simulink model "igct_diode"  (R2023b)
settings: Solver=VariableStepAuto  StartTime=0.0  StopTime=10.0  RelTol=1e-3
values from neighbouring files (symbols this model uses):
  temp_init = 40    [power_sysinit.m]
  Ts1 = 1e-6    (= 1e-06)    [power_sysinit.m]
  Ts2 = 500E-6    (= 0.0005)    [power_sysinit.m]
  Udc = 2500    [power_sysinit.m]
undefined symbols (not defined in the file or in its folder): DIODE_204520, DIODE_344520, DIODE_364520, DIODE_364521, DIODE_D1031SH, DIODE_D1331SH, IGCT_364520_36, IGCT_364521_36, IGCT_654522_6, magnitude, Rch_DIODE, Rch_tau_DIODE, Rjc1_DIODE, Rjc1_tau_DIODE, Rjc2_DIODE, Rjc2_tau_DIODE, Rjc3_DIODE, Rjc3_tau_DIODE, Rth_h, Rth_h_tau
libraries: spsMeanLib x304, simulink x52, spsRMSLib x52
(part 7 of 11)

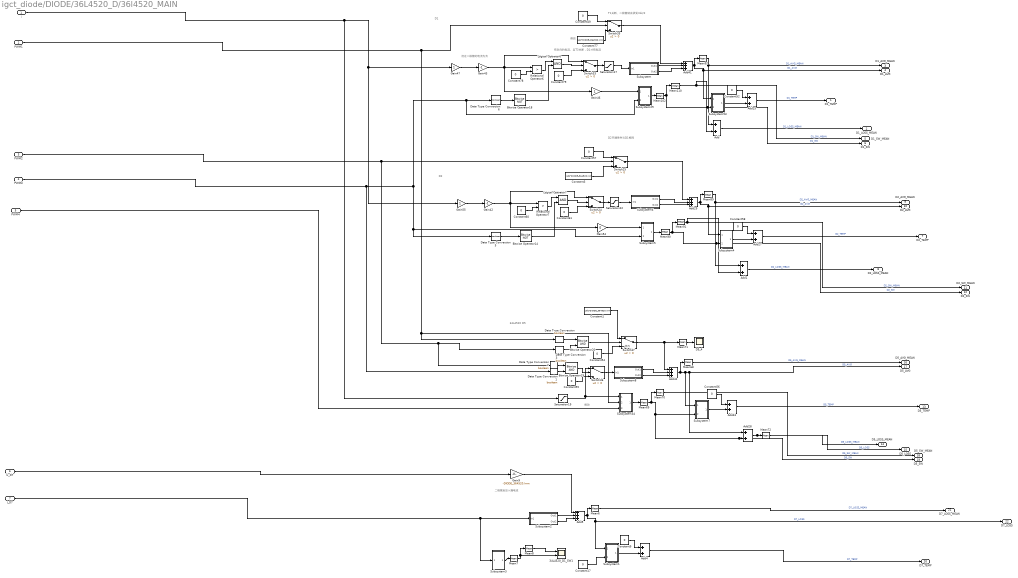
== system igct_diode/DIODE/36L4520_D/36l4520_MAIN ==
  note: 修改
  note: 34L4520 D5
  note: 修改
  note: 二极管反压×漏电流
  note: D2
  note: 有负向的电流、且T3关断，D1才有电流
  note: 修改
  note: 流过二极管的电流为负
  note: D2开通条件与D1相同
  note: T1关断、二极管就会承受Vdc/2
  note: D1
  i : Inport
  PWM1 : Inport  Port=2
  PWM2 : Inport  Port=3
  PWM3 : Inport  Port=4
  PWM4 : Inport  Port=5
  U_D7 : Inport  Port=6
  I_D7 : Inport  Port=7
  34L4520_D1_SW1 : Scope  NumInputPorts=2
  Add{,1,4,25,27..28,43} (7 alike) : Sum
  Add{5,29,41..42} (4 alike) : Sum  Inputs=+++
  Bitwise Operator14 : simulink/Logic and Bit Operations/Bitwise Operator  logicop=NOT  UseBitMask=off  BitMask=bin2dec('11011001')  BitMaskRealWorld=Stored Integer
  Bitwise Operator18 : simulink/Logic and Bit Operations/Bitwise Operator  logicop=NOT  UseBitMask=off  BitMask=bin2dec('11011001')  BitMaskRealWorld=Stored Integer
  Bitwise Operator19 : simulink/Logic and Bit Operations/Bitwise Operator  logicop=AND  UseBitMask=off  NumInputPorts=2  BitMask=bin2dec('11011001')  BitMaskRealWorld=Stored Integer
  Bitwise Operator20 : simulink/Logic and Bit Operations/Bitwise Operator  logicop=AND  UseBitMask=off  NumInputPorts=2  BitMask=bin2dec('11011001')  BitMaskRealWorld=Stored Integer
  Constant1 : Constant  Value=Udc*DIODE_364520.Irrm
  Constant{9,17,49,52,54..58,60..61,78..79} (13 alike) : Constant  Value=0
  Constant3 : Constant  Value=Udc*DIODE_364520.Irrm
  Constant77 : Constant  Value=Udc*DIODE_364520.Irrm
  D5_4 : Scope
  Data Type Conversion{,1..3,5..6} (6 alike) : DataTypeConversion  OutDataTypeStr=boolean  SaturateOnIntegerOverflow=off  RndMeth=Floor
  Gain42 : Gain  Gain=-1
  Gain43 : Gain  Gain=-1
  Gain46 : Gain
  Gain47 : Gain
  Gain54 : Gain  Gain=0
  Gain55 : Gain
  Gain9 : Gain  Gain=-DIODE_364520.Irrm
  Logical Operator6 : Logic  AllPortsSameDT=off  OutDataTypeStr=boolean
  Logical Operator7 : Logic  AllPortsSameDT=off  OutDataTypeStr=boolean
  Mean{7,69,90,102} (4 alike) : spsMeanLib/Mean  Freq=2000  Vinit=0  Ts=Ts1
  Mean{6,8,68,70,72,91..92,110} (8 alike) : spsMeanLib/Mean  Freq=f  Vinit=0  Ts=Ts1
  Mean71 : spsMeanLib/Mean  Freq=1  Vinit=0  Ts=Ts1
  Mean89 : spsMeanLib/Mean  Freq=f  Vinit=0  Ts=1e-6
  Relational Operator6 : RelationalOperator  Operator=>  OutDataTypeStr=boolean  RndMeth=Simplest  InputSameDT=off
  Relational Operator7 : RelationalOperator  Operator=>  OutDataTypeStr=boolean  RndMeth=Simplest  InputSameDT=off
  Saturation17 : Saturate  UpperLimit=5500  LowerLimit=0
  Saturation19 : Saturate  UpperLimit=5000  LowerLimit=0
  Saturation22 : Saturate  UpperLimit=5500  LowerLimit=0
  Subsystem : Subsystem
  Subsystem1 : Subsystem
  Subsystem2 : Subsystem
  Subsystem29 : Subsystem
  Subsystem3 : Subsystem
  Subsystem34 : Subsystem
  Subsystem4 : Subsystem
  Subsystem5 : Subsystem
  Subsystem53 : Subsystem
  Subsystem6 : Subsystem
  Subsystem7 : Subsystem
  Subsystem8 : Subsystem
  Switch{24..25,33,35..37} (6 alike) : Switch  Criteria=u2 > Threshold  SaturateOnIntegerOverflow=off  InputSameDT=off
  D1_TEMP : Outport
  D1_LOSS_MEAN : Outport  Port=2
  D1_AVG_MEAN : Outport  Port=3
  D1_AVG : Outport  Port=4
  D1_SW_MEAN : Outport  Port=5
  D1_SW : Outport  Port=6
  D2_TEMP : Outport  Port=7
  D2_LOSS_MEAN : Outport  Port=8
  D2_AVG_MEAN : Outport  Port=9
  D2_AVG : Outport  Port=10
  D2_SW_MEAN : Outport  Port=11
  D2_SW : Outport  Port=12
  D5_TEMP : Outport  Port=13
  D5_LOSS_MEAN : Outport  Port=14
  D5_LOSS : Outport  Port=15
  D5_AVG_MEAN : Outport  Port=16
  D5_AVG : Outport  Port=17
  D5_SW_MEAN : Outport  Port=18
  D5_SW : Outport  Port=19
  D7_TEMP : Outport  Port=20
  D7_LOSS_MEAN : Outport  Port=21
  D7_LOSS : Outport  Port=22
  wires:
  Add1/1 -> D2_LOSS_MEAN/1  "D2_LOSS_MEAN"
  Add/1 -> D1_LOSS_MEAN/1  "D1_LOSS_MEAN"
  Add27/1 -> D2_TEMP/1  "D2_TEMP"
  Add4/1 -> D7_TEMP/1  "D7_TEMP"
  U_D7/1 -> Gain9/1
  Mean70/1 -> D5_SW_MEAN/1  "D5_SW_MEAN"
  Subsystem/2(Out2) -> Add41/3
  Saturation17/1 -> Subsystem/1(In1)
  Constant60/1 -> Relational Operator7/2
  Gain47/1 -> Gain43/1
  Data Type Conversion6/1 -> Bitwise Operator18/1
  Constant78/1 -> Relational Operator6/2
  Data Type Conversion5/1 -> Bitwise Operator14/1
  Constant57/1 -> Switch25/1
  Bitwise Operator18/1 -> Logical Operator6/2
  Constant77/1 -> Switch35/3
  Mean89/1 -> Add1/1, D2_AVG_MEAN/1  "D2_AVG_MEAN"
  Subsystem53/1(Out1) -> Add25/2
  Constant52/1 -> Add25/1
  Add43/1 -> D5_TEMP/1  "D5_TEMP"
  Logical Operator6/1 -> Switch33/2
  Constant49/1 -> Switch35/1
  Gain46/1 -> Subsystem29/1(In1)
  Gain42/1 -> Switch24/1, Gain54/1, Relational Operator7/1
  Switch24/1 -> Saturation22/1
  Constant79/1 -> Switch33/3
  Mean92/1 -> Add/1, D1_AVG_MEAN/1  "D1_AVG_MEAN"
  Switch35/1 -> Add41/1
  Switch25/1 -> Add29/1
  Mean6/1 -> D7_LOSS_MEAN/1  "D7_LOSS_MEAN"
  Gain43/1 -> Relational Operator6/1, Gain46/1, Switch33/1
  Add41/1 -> Mean92/1, Subsystem53/1(In1), D1_AVG/1  "D1_AVG"
  Subsystem4/1(Out1) -> Add27/2
  Data Type Conversion2/1 -> Bitwise Operator19/1
  Constant55/1 -> Switch36/3
  Subsystem3/1(Out1) -> Mean7/1
  Subsystem6/2(Out2) -> Add29/3
  Switch37/1 -> Add42/1, Mean71/1
  Constant54/1 -> Switch37/3
  Subsystem7/1(Out1) -> Add43/2
  Subsystem/1(Out1) -> Add41/2
  Gain9/1 -> Add5/1
  Constant58/1 -> Add27/1
  Subsystem8/1(Out1) -> Add42/2
  Mean8/1 -> 34L4520_D1_SW1/1
  Gain54/1 -> Subsystem5/1(In1)
  Mean102/1 -> Subsystem53/2(In2), D1_SW/1, Mean110/1  "D1_SW"
  Subsystem1/1(Out1) -> Add4/2
  Subsystem5/1(Out1) -> Mean90/1
  I_D7/1 -> Subsystem2/1(In1), Subsystem3/1(In1)
  Logical Operator7/1 -> Switch24/2
  Add5/1 -> Subsystem1/1(In1), D7_LOSS/1, Mean6/1  "D7_LOSS"
  Data Type Conversion3/1 -> Bitwise Operator20/2
  Mean7/1 -> Mean8/1, 34L4520_D1_SW1/2
  Relational Operator7/1 -> Logical Operator7/1
  Constant17/1 -> Subsystem1/2(In2)
  Subsystem2/2(Out2) -> Add5/3
  Add25/1 -> D1_TEMP/1  "D1_TEMP"
  Mean69/1 -> Mean70/1, Subsystem7/2(In2), Add28/2, D5_SW/1  "D5_SW"
  Bitwise Operator20/1 -> Switch37/2
  PWM4/1 -> Subsystem34/3(In3)
  Bitwise Operator19/1 -> Switch36/2
  Mean91/1 -> Add1/2, D2_SW_MEAN/1  "D2_SW_MEAN"
  PWM2/1 -> Switch25/2, Data Type Conversion3/1, Data Type Conversion2/1
  Switch33/1 -> Saturation17/1
  Mean110/1 -> Add/2, D1_SW_MEAN/1  "D1_SW_MEAN"
  Mean71/1 -> D5_4/1
  PWM3/1 -> Subsystem5/2(In2), Data Type Conversion5/1, Subsystem29/2(In2), Data Type Conversion6/1, Data Type Conversion1/1
  i/1 -> Gain47/1, Gain55/1, Saturation19/1
  Subsystem6/1(Out1) -> Add29/2
  Data Type Conversion1/1 -> Bitwise Operator19/2
  Constant61/1 -> Switch24/3
  Mean72/1 -> D5_LOSS_MEAN/1  "D5_LOSS_MEAN"
  Mean90/1 -> Mean91/1, D2_SW/1, Subsystem4/2(In2)  "D2_SW"
  PWM1/1 -> Switch35/2, Data Type Conversion/1, Subsystem34/2(In2)
  Relational Operator6/1 -> Logical Operator6/1
  Mean68/1 -> D5_AVG_MEAN/1  "D5_AVG_MEAN"
  Saturation19/1 -> Subsystem34/1(In1), Switch36/1
  Switch36/1 -> Subsystem8/1(In1)
  Subsystem8/2(Out2) -> Add42/3
  Gain55/1 -> Gain42/1
  Constant3/1 -> Switch25/3
  Constant9/1 -> Add4/1
  Subsystem34/1(Out1) -> Mean69/1
  Add42/1 -> Mean68/1, Subsystem7/1(In1), Add28/1, D5_AVG/1  "D5_AVG"
  Data Type Conversion/1 -> Bitwise Operator20/1
  Bitwise Operator14/1 -> Logical Operator7/2
  Saturation22/1 -> Subsystem6/1(In1)
  Add29/1 -> Subsystem4/1(In1), D2_AVG/1, Mean89/1  "D2_AVG"
  Constant1/1 -> Switch37/1
  Constant56/1 -> Add43/1
  Subsystem2/1(Out1) -> Add5/2
  Subsystem29/1(Out1) -> Mean102/1
  Add28/1 -> Mean72/1, D5_LOSS/1  "D5_LOSS"

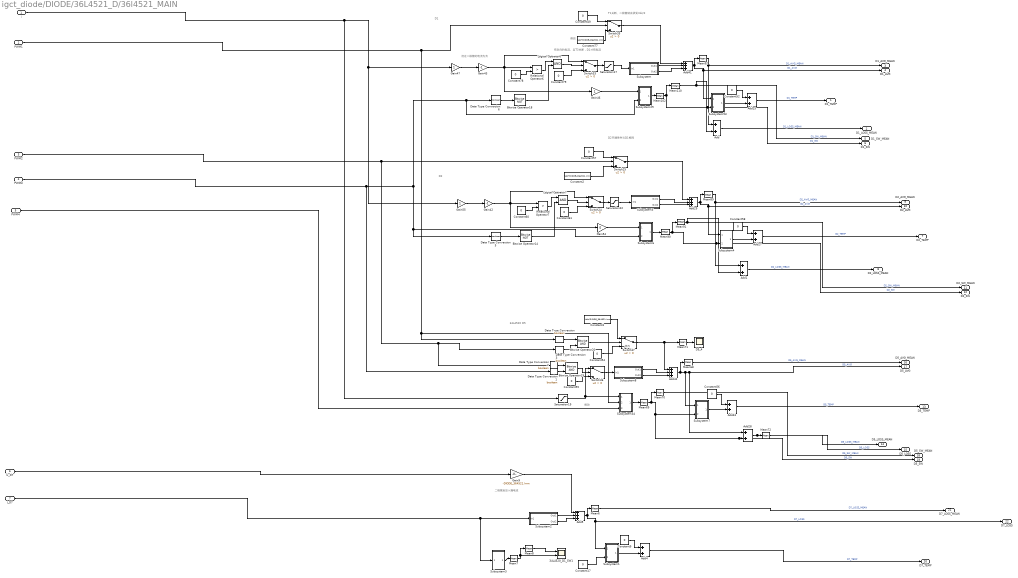
== system igct_diode/DIODE/36L4521_D/36l4521_MAIN ==
  note: D1
  note: T1关断、二极管就会承受Vdc/2
  note: D2开通条件与D1相同
  note: 流过二极管的电流为负
  note: 修改
  note: 有负向的电流、且T3关断，D1才有电流
  note: D2
  note: 二极管反压×漏电流
  note: 修改
  note: 34L4520 D5
  note: 修改
  i : Inport
  PWM1 : Inport  Port=2
  PWM2 : Inport  Port=3
  PWM3 : Inport  Port=4
  PWM4 : Inport  Port=5
  U_D7 : Inport  Port=6
  I_D7 : Inport  Port=7
  34L4520_D1_SW1 : Scope  NumInputPorts=2
  Add{,1,4,25,27..28,43} (7 alike) : Sum
  Add{5,29,41..42} (4 alike) : Sum  Inputs=+++
  Bitwise Operator14 : simulink/Logic and Bit Operations/Bitwise Operator  logicop=NOT  UseBitMask=off  BitMask=bin2dec('11011001')  BitMaskRealWorld=Stored Integer
  Bitwise Operator18 : simulink/Logic and Bit Operations/Bitwise Operator  logicop=NOT  UseBitMask=off  BitMask=bin2dec('11011001')  BitMaskRealWorld=Stored Integer
  Bitwise Operator19 : simulink/Logic and Bit Operations/Bitwise Operator  logicop=AND  UseBitMask=off  NumInputPorts=2  BitMask=bin2dec('11011001')  BitMaskRealWorld=Stored Integer
  Bitwise Operator20 : simulink/Logic and Bit Operations/Bitwise Operator  logicop=AND  UseBitMask=off  NumInputPorts=2  BitMask=bin2dec('11011001')  BitMaskRealWorld=Stored Integer
  Constant{9,17,49,52,54..58,60..61,78..79} (13 alike) : Constant  Value=0
  Constant2 : Constant  Value=Udc*DIODE_364521.Irrm
  Constant3 : Constant  Value=Udc*DIODE_364521.Irrm
  Constant77 : Constant  Value=Udc*DIODE_364521.Irrm
  D5_4 : Scope
  Data Type Conversion{,1..3,5..6} (6 alike) : DataTypeConversion  OutDataTypeStr=boolean  SaturateOnIntegerOverflow=off  RndMeth=Floor
  Gain42 : Gain  Gain=-1
  Gain43 : Gain  Gain=-1
  Gain46 : Gain
  Gain47 : Gain
  Gain54 : Gain  Gain=0
  Gain55 : Gain
  Gain9 : Gain  Gain=-DIODE_364521.Irrm
  Logical Operator6 : Logic  AllPortsSameDT=off  OutDataTypeStr=boolean
  Logical Operator7 : Logic  AllPortsSameDT=off  OutDataTypeStr=boolean
  Mean{7,69,90,102} (4 alike) : spsMeanLib/Mean  Freq=2000  Vinit=0  Ts=Ts1
  Mean{6,8,68,70,72,91..92,110} (8 alike) : spsMeanLib/Mean  Freq=f  Vinit=0  Ts=Ts1
  Mean71 : spsMeanLib/Mean  Freq=1  Vinit=0  Ts=Ts1
  Mean89 : spsMeanLib/Mean  Freq=f  Vinit=0  Ts=1e-6
  Relational Operator6 : RelationalOperator  Operator=>  OutDataTypeStr=boolean  RndMeth=Simplest  InputSameDT=off
  Relational Operator7 : RelationalOperator  Operator=>  OutDataTypeStr=boolean  RndMeth=Simplest  InputSameDT=off
  Saturation17 : Saturate  UpperLimit=5500  LowerLimit=0
  Saturation19 : Saturate  UpperLimit=5000  LowerLimit=0
  Saturation22 : Saturate  UpperLimit=5500  LowerLimit=0
  Subsystem : Subsystem
  Subsystem1 : Subsystem
  Subsystem2 : Subsystem
  Subsystem29 : Subsystem
  Subsystem3 : Subsystem
  Subsystem34 : Subsystem
  Subsystem4 : Subsystem
  Subsystem5 : Subsystem
  Subsystem53 : Subsystem
  Subsystem6 : Subsystem
  Subsystem7 : Subsystem
  Subsystem8 : Subsystem
  Switch{24..25,33,35..37} (6 alike) : Switch  Criteria=u2 > Threshold  SaturateOnIntegerOverflow=off  InputSameDT=off
  D1_TEMP : Outport
  D1_LOSS_MEAN : Outport  Port=2
  D1_AVG_MEAN : Outport  Port=3
  D1_AVG : Outport  Port=4
  D1_SW_MEAN : Outport  Port=5
  D1_SW : Outport  Port=6
  D2_TEMP : Outport  Port=7
  D2_LOSS_MEAN : Outport  Port=8
  D2_AVG_MEAN : Outport  Port=9
  D2_AVG : Outport  Port=10
  D2_SW_MEAN : Outport  Port=11
  D2_SW : Outport  Port=12
  D5_TEMP : Outport  Port=13
  D5_LOSS_MEAN : Outport  Port=14
  D5_LOSS : Outport  Port=15
  D5_AVG_MEAN : Outport  Port=16
  D5_AVG : Outport  Port=17
  D5_SW_MEAN : Outport  Port=18
  D5_SW : Outport  Port=19
  D7_TEMP : Outport  Port=20
  D7_LOSS_MEAN : Outport  Port=21
  D7_LOSS : Outport  Port=22
  wires:
  Add28/1 -> D5_LOSS/1, Mean72/1  "D5_LOSS"
  Subsystem29/1(Out1) -> Mean102/1
  Subsystem2/1(Out1) -> Add5/2
  Constant56/1 -> Add43/1
  Constant3/1 -> Switch37/1
  Add29/1 -> Mean89/1, Subsystem4/1(In1), D2_AVG/1  "D2_AVG"
  Saturation22/1 -> Subsystem5/1(In1)
  Bitwise Operator14/1 -> Logical Operator7/2
  Data Type Conversion/1 -> Bitwise Operator20/1
  Add42/1 -> Subsystem7/1(In1), D5_AVG/1, Add28/1, Mean68/1  "D5_AVG"
  Subsystem34/1(Out1) -> Mean69/1
  Constant9/1 -> Add4/1
  Constant2/1 -> Switch25/3
  Gain55/1 -> Gain42/1
  Subsystem8/2(Out2) -> Add42/3
  Switch36/1 -> Subsystem8/1(In1)
  Saturation19/1 -> Switch36/1, Subsystem34/1(In1)
  Mean68/1 -> D5_AVG_MEAN/1  "D5_AVG_MEAN"
  Relational Operator6/1 -> Logical Operator6/1
  PWM1/1 -> Subsystem34/2(In2), Data Type Conversion/1, Switch35/2
  Mean90/1 -> D2_SW/1, Subsystem4/2(In2), Mean91/1  "D2_SW"
  Mean72/1 -> D5_LOSS_MEAN/1  "D5_LOSS_MEAN"
  Constant61/1 -> Switch24/3
  Data Type Conversion1/1 -> Bitwise Operator19/2
  Subsystem5/1(Out1) -> Add29/2
  i/1 -> Saturation19/1, Gain55/1, Gain47/1
  PWM3/1 -> Data Type Conversion1/1, Data Type Conversion6/1, Subsystem29/2(In2), Subsystem6/2(In2), Data Type Conversion5/1
  Mean71/1 -> D5_4/1
  Mean110/1 -> D1_SW_MEAN/1, Add/2  "D1_SW_MEAN"
  Switch33/1 -> Saturation17/1
  PWM2/1 -> Data Type Conversion2/1, Data Type Conversion3/1, Switch25/2
  Mean91/1 -> D2_SW_MEAN/1, Add1/2  "D2_SW_MEAN"
  Bitwise Operator19/1 -> Switch36/2
  PWM4/1 -> Subsystem34/3(In3)
  Bitwise Operator20/1 -> Switch37/2
  Mean69/1 -> Subsystem7/2(In2), D5_SW/1, Add28/2, Mean70/1  "D5_SW"
  Add25/1 -> D1_TEMP/1  "D1_TEMP"
  Subsystem2/2(Out2) -> Add5/3
  Constant17/1 -> Subsystem1/2(In2)
  Relational Operator7/1 -> Logical Operator7/1
  Mean7/1 -> 34L4520_D1_SW1/2, Mean8/1
  Data Type Conversion3/1 -> Bitwise Operator20/2
  Add5/1 -> Mean6/1, Subsystem1/1(In1), D7_LOSS/1  "D7_LOSS"
  Logical Operator7/1 -> Switch24/2
  I_D7/1 -> Subsystem2/1(In1), Subsystem3/1(In1)
  Subsystem6/1(Out1) -> Mean90/1
  Subsystem1/1(Out1) -> Add4/2
  Mean102/1 -> Mean110/1, D1_SW/1, Subsystem53/2(In2)  "D1_SW"
  Gain54/1 -> Subsystem6/1(In1)
  Mean8/1 -> 34L4520_D1_SW1/1
  Subsystem8/1(Out1) -> Add42/2
  Constant58/1 -> Add27/1
  Gain9/1 -> Add5/1
  Subsystem/1(Out1) -> Add41/2
  Subsystem7/1(Out1) -> Add43/2
  Constant54/1 -> Switch37/3
  Switch37/1 -> Mean71/1, Add42/1
  Subsystem5/2(Out2) -> Add29/3
  Subsystem3/1(Out1) -> Mean7/1
  Constant55/1 -> Switch36/3
  Data Type Conversion2/1 -> Bitwise Operator19/1
  Subsystem4/1(Out1) -> Add27/2
  Add41/1 -> D1_AVG/1, Subsystem53/1(In1), Mean92/1  "D1_AVG"
  Gain43/1 -> Switch33/1, Gain46/1, Relational Operator6/1
  Mean6/1 -> D7_LOSS_MEAN/1  "D7_LOSS_MEAN"
  Switch25/1 -> Add29/1
  Switch35/1 -> Add41/1
  Mean92/1 -> D1_AVG_MEAN/1, Add/1  "D1_AVG_MEAN"
  Constant79/1 -> Switch33/3
  Switch24/1 -> Saturation22/1
  Gain42/1 -> Relational Operator7/1, Gain54/1, Switch24/1
  Gain46/1 -> Subsystem29/1(In1)
  Constant49/1 -> Switch35/1
  Logical Operator6/1 -> Switch33/2
  Add43/1 -> D5_TEMP/1  "D5_TEMP"
  Constant52/1 -> Add25/1
  Subsystem53/1(Out1) -> Add25/2
  Mean89/1 -> D2_AVG_MEAN/1, Add1/1  "D2_AVG_MEAN"
  Constant77/1 -> Switch35/3
  Bitwise Operator18/1 -> Logical Operator6/2
  Constant57/1 -> Switch25/1
  Data Type Conversion5/1 -> Bitwise Operator14/1
  Constant78/1 -> Relational Operator6/2
  Data Type Conversion6/1 -> Bitwise Operator18/1
  Gain47/1 -> Gain43/1
  Constant60/1 -> Relational Operator7/2
  Saturation17/1 -> Subsystem/1(In1)
  Subsystem/2(Out2) -> Add41/3
  Mean70/1 -> D5_SW_MEAN/1  "D5_SW_MEAN"
  U_D7/1 -> Gain9/1
  Add4/1 -> D7_TEMP/1  "D7_TEMP"
  Add27/1 -> D2_TEMP/1  "D2_TEMP"
  Add/1 -> D1_LOSS_MEAN/1  "D1_LOSS_MEAN"
  Add1/1 -> D2_LOSS_MEAN/1  "D2_LOSS_MEAN"

== system igct_diode/DIODE/D1031SH/D1031SH_MAIN ==
  note: D1
  note: T1关断、二极管就会承受Vdc/2
  note: D2开通条件与D1相同
  note: 流过二极管的电流为负
  note: 修改
  note: 有负向的电流、且T3关断，D1才有电流
  note: D2
  note: 二极管反压×漏电流
  note: 修改
  note: 34L4520 D5
  note: 修改
  i : Inport
  PWM1 : Inport  Port=2
  PWM2 : Inport  Port=3
  PWM3 : Inport  Port=4
  PWM4 : Inport  Port=5
  U_D7 : Inport  Port=6
  I_D7 : Inport  Port=7
  34L4520_D1_SW1 : Scope  NumInputPorts=2
  Add{,1,4,25,27..28,43} (7 alike) : Sum
  Add{5,29,41..42} (4 alike) : Sum  Inputs=+++
  Bitwise Operator14 : simulink/Logic and Bit Operations/Bitwise Operator  logicop=NOT  UseBitMask=off  BitMask=bin2dec('11011001')  BitMaskRealWorld=Stored Integer
  Bitwise Operator18 : simulink/Logic and Bit Operations/Bitwise Operator  logicop=NOT  UseBitMask=off  BitMask=bin2dec('11011001')  BitMaskRealWorld=Stored Integer
  Bitwise Operator19 : simulink/Logic and Bit Operations/Bitwise Operator  logicop=AND  UseBitMask=off  NumInputPorts=2  BitMask=bin2dec('11011001')  BitMaskRealWorld=Stored Integer
  Bitwise Operator20 : simulink/Logic and Bit Operations/Bitwise Operator  logicop=AND  UseBitMask=off  NumInputPorts=2  BitMask=bin2dec('11011001')  BitMaskRealWorld=Stored Integer
  Constant1 : Constant  Value=Udc*DIODE_204520.Irrm
  Constant{9,17,49,52,54..58,60..61,78..79} (13 alike) : Constant  Value=0
  Constant2 : Constant  Value=Udc*DIODE_D1031SH.Irrm
  Constant77 : Constant  Value=Udc*DIODE_D1031SH.Irrm
  D5_4 : Scope
  Data Type Conversion{,1..3,5..6} (6 alike) : DataTypeConversion  OutDataTypeStr=boolean  SaturateOnIntegerOverflow=off  RndMeth=Floor
  Gain42 : Gain  Gain=-1
  Gain43 : Gain  Gain=-1
  Gain46 : Gain
  Gain47 : Gain
  Gain54 : Gain  Gain=0
  Gain55 : Gain
  Gain9 : Gain  Gain=-DIODE_D1031SH.Irrm
  Logical Operator6 : Logic  AllPortsSameDT=off  OutDataTypeStr=boolean
  Logical Operator7 : Logic  AllPortsSameDT=off  OutDataTypeStr=boolean
  Mean{7,69,90,102} (4 alike) : spsMeanLib/Mean  Freq=2000  Vinit=0  Ts=Ts1
  Mean{6,8,68,70,72,91..92,110} (8 alike) : spsMeanLib/Mean  Freq=f  Vinit=0  Ts=Ts1
  Mean71 : spsMeanLib/Mean  Freq=1  Vinit=0  Ts=Ts1
  Mean89 : spsMeanLib/Mean  Freq=f  Vinit=0  Ts=1e-6
  Relational Operator6 : RelationalOperator  Operator=>  OutDataTypeStr=boolean  RndMeth=Simplest  InputSameDT=off
  Relational Operator7 : RelationalOperator  Operator=>  OutDataTypeStr=boolean  RndMeth=Simplest  InputSameDT=off
  Saturation17 : Saturate  UpperLimit=5500  LowerLimit=0
  Saturation19 : Saturate  UpperLimit=5000  LowerLimit=0
  Saturation22 : Saturate  UpperLimit=5500  LowerLimit=0
  Subsystem : Subsystem
  Subsystem1 : Subsystem
  Subsystem2 : Subsystem
  Subsystem29 : Subsystem
  Subsystem3 : Subsystem
  Subsystem34 : Subsystem
  Subsystem4 : Subsystem
  Subsystem5 : Subsystem
  Subsystem53 : Subsystem
  Subsystem6 : Subsystem
  Subsystem7 : Subsystem
  Subsystem9 : Subsystem
  Switch{24..25,33,35..37} (6 alike) : Switch  Criteria=u2 > Threshold  SaturateOnIntegerOverflow=off  InputSameDT=off
  D1_TEMP : Outport
  D1_LOSS_MEAN : Outport  Port=2
  D1_AVG_MEAN : Outport  Port=3
  D1_AVG : Outport  Port=4
  D1_SW_MEAN : Outport  Port=5
  D1_SW : Outport  Port=6
  D2_TEMP : Outport  Port=7
  D2_LOSS_MEAN : Outport  Port=8
  D2_AVG_MEAN : Outport  Port=9
  D2_AVG : Outport  Port=10
  D2_SW_MEAN : Outport  Port=11
  D2_SW : Outport  Port=12
  D5_TEMP : Outport  Port=13
  D5_LOSS_MEAN : Outport  Port=14
  D5_LOSS : Outport  Port=15
  D5_AVG_MEAN : Outport  Port=16
  D5_AVG : Outport  Port=17
  D5_SW_MEAN : Outport  Port=18
  D5_SW : Outport  Port=19
  D7_TEMP : Outport  Port=20
  D7_LOSS_MEAN : Outport  Port=21
  D7_LOSS : Outport  Port=22
  wires:
  Add28/1 -> D5_LOSS/1, Mean72/1  "D5_LOSS"
  Subsystem29/1(Out1) -> Mean102/1
  Subsystem7/1(Out1) -> Add5/2
  Constant56/1 -> Add43/1
  Constant1/1 -> Switch37/1
  Add29/1 -> Mean89/1, Subsystem4/1(In1), D2_AVG/1  "D2_AVG"
  Saturation22/1 -> Subsystem2/1(In1)
  Bitwise Operator14/1 -> Logical Operator7/2
  Data Type Conversion/1 -> Bitwise Operator20/1
  Add42/1 -> Subsystem6/1(In1), D5_AVG/1, Add28/1, Mean68/1  "D5_AVG"
  Subsystem34/1(Out1) -> Mean69/1
  Constant9/1 -> Add4/1
  Constant2/1 -> Switch25/3
  Gain55/1 -> Gain42/1
  Subsystem5/2(Out2) -> Add42/3
  Switch36/1 -> Subsystem5/1(In1)
  Saturation19/1 -> Switch36/1, Subsystem34/1(In1)
  Mean68/1 -> D5_AVG_MEAN/1  "D5_AVG_MEAN"
  Relational Operator6/1 -> Logical Operator6/1
  PWM1/1 -> Subsystem34/2(In2), Data Type Conversion/1, Switch35/2
  Mean90/1 -> Subsystem4/2(In2), D2_SW/1, Mean91/1  "D2_SW"
  Mean72/1 -> D5_LOSS_MEAN/1  "D5_LOSS_MEAN"
  Constant61/1 -> Switch24/3
  Data Type Conversion1/1 -> Bitwise Operator19/2
  Subsystem2/1(Out1) -> Add29/2
  i/1 -> Saturation19/1, Gain55/1, Gain47/1
  PWM3/1 -> Data Type Conversion1/1, Data Type Conversion6/1, Subsystem29/2(In2), Subsystem9/2(In2), Data Type Conversion5/1
  Mean71/1 -> D5_4/1
  Mean110/1 -> D1_SW_MEAN/1, Add/2  "D1_SW_MEAN"
  Switch33/1 -> Saturation17/1
  PWM2/1 -> Data Type Conversion2/1, Data Type Conversion3/1, Switch25/2
  Mean91/1 -> D2_SW_MEAN/1, Add1/2  "D2_SW_MEAN"
  Bitwise Operator19/1 -> Switch36/2
  PWM4/1 -> Subsystem34/3(In3)
  Bitwise Operator20/1 -> Switch37/2
  Mean69/1 -> Subsystem6/2(In2), D5_SW/1, Add28/2, Mean70/1  "D5_SW"
  Add25/1 -> D1_TEMP/1  "D1_TEMP"
  Subsystem7/2(Out2) -> Add5/3
  Constant17/1 -> Subsystem1/2(In2)
  Relational Operator7/1 -> Logical Operator7/1
  Mean7/1 -> 34L4520_D1_SW1/2, Mean8/1
  Data Type Conversion3/1 -> Bitwise Operator20/2
  Add5/1 -> Mean6/1, Subsystem1/1(In1), D7_LOSS/1  "D7_LOSS"
  Logical Operator7/1 -> Switch24/2
  I_D7/1 -> Subsystem7/1(In1), Subsystem3/1(In1)
  Subsystem9/1(Out1) -> Mean90/1
  Subsystem1/1(Out1) -> Add4/2
  Mean102/1 -> Mean110/1, D1_SW/1, Subsystem53/2(In2)  "D1_SW"
  Gain54/1 -> Subsystem9/1(In1)
  Mean8/1 -> 34L4520_D1_SW1/1
  Subsystem5/1(Out1) -> Add42/2
  Constant58/1 -> Add27/1
  Gain9/1 -> Add5/1
  Subsystem/1(Out1) -> Add41/2
  Subsystem6/1(Out1) -> Add43/2
  Constant54/1 -> Switch37/3
  Switch37/1 -> Mean71/1, Add42/1
  Subsystem2/2(Out2) -> Add29/3
  Subsystem3/1(Out1) -> Mean7/1
  Constant55/1 -> Switch36/3
  Data Type Conversion2/1 -> Bitwise Operator19/1
  Subsystem4/1(Out1) -> Add27/2
  Add41/1 -> D1_AVG/1, Subsystem53/1(In1), Mean92/1  "D1_AVG"
  Gain43/1 -> Switch33/1, Gain46/1, Relational Operator6/1
  Mean6/1 -> D7_LOSS_MEAN/1  "D7_LOSS_MEAN"
  Switch25/1 -> Add29/1
  Switch35/1 -> Add41/1
  Mean92/1 -> D1_AVG_MEAN/1, Add/1  "D1_AVG_MEAN"
  Constant79/1 -> Switch33/3
  Switch24/1 -> Saturation22/1
  Gain42/1 -> Relational Operator7/1, Gain54/1, Switch24/1
  Gain46/1 -> Subsystem29/1(In1)
  Constant49/1 -> Switch35/1
  Logical Operator6/1 -> Switch33/2
  Add43/1 -> D5_TEMP/1  "D5_TEMP"
  Constant52/1 -> Add25/1
  Subsystem53/1(Out1) -> Add25/2
  Mean89/1 -> D2_AVG_MEAN/1, Add1/1  "D2_AVG_MEAN"
  Constant77/1 -> Switch35/3
  Bitwise Operator18/1 -> Logical Operator6/2
  Constant57/1 -> Switch25/1
  Data Type Conversion5/1 -> Bitwise Operator14/1
  Constant78/1 -> Relational Operator6/2
  Data Type Conversion6/1 -> Bitwise Operator18/1
  Gain47/1 -> Gain43/1
  Constant60/1 -> Relational Operator7/2
  Saturation17/1 -> Subsystem/1(In1)
  Subsystem/2(Out2) -> Add41/3
  Mean70/1 -> D5_SW_MEAN/1  "D5_SW_MEAN"
  U_D7/1 -> Gain9/1
  Add4/1 -> D7_TEMP/1  "D7_TEMP"
  Add27/1 -> D2_TEMP/1  "D2_TEMP"
  Add/1 -> D1_LOSS_MEAN/1  "D1_LOSS_MEAN"
  Add1/1 -> D2_LOSS_MEAN/1  "D2_LOSS_MEAN"

== system igct_diode/DIODE/D1331SH/D1331SH_MAIN ==
  note: 修改
  note: 34L4520 D5
  note: 修改
  note: 二极管反压×漏电流
  note: D2
  note: 有负向的电流、且T3关断，D1才有电流
  note: 修改
  note: 流过二极管的电流为负
  note: D2开通条件与D1相同
  note: T1关断、二极管就会承受Vdc/2
  note: D1
  i : Inport
  PWM1 : Inport  Port=2
  PWM2 : Inport  Port=3
  PWM3 : Inport  Port=4
  PWM4 : Inport  Port=5
  U_D7 : Inport  Port=6
  I_D7 : Inport  Port=7
  34L4520_D1_SW1 : Scope  NumInputPorts=2
  Add{,1,4,25,27..28,43} (7 alike) : Sum
  Add{5,29,41..42} (4 alike) : Sum  Inputs=+++
  Bitwise Operator14 : simulink/Logic and Bit Operations/Bitwise Operator  logicop=NOT  UseBitMask=off  BitMask=bin2dec('11011001')  BitMaskRealWorld=Stored Integer
  Bitwise Operator18 : simulink/Logic and Bit Operations/Bitwise Operator  logicop=NOT  UseBitMask=off  BitMask=bin2dec('11011001')  BitMaskRealWorld=Stored Integer
  Bitwise Operator19 : simulink/Logic and Bit Operations/Bitwise Operator  logicop=AND  UseBitMask=off  NumInputPorts=2  BitMask=bin2dec('11011001')  BitMaskRealWorld=Stored Integer
  Bitwise Operator20 : simulink/Logic and Bit Operations/Bitwise Operator  logicop=AND  UseBitMask=off  NumInputPorts=2  BitMask=bin2dec('11011001')  BitMaskRealWorld=Stored Integer
  Constant{9,17,49,52,54..58,60..61,78..79} (13 alike) : Constant  Value=0
  Constant2 : Constant  Value=Udc*DIODE_D1331SH.Irrm
  Constant3 : Constant  Value=Udc*DIODE_D1331SH.Irrm
  Constant77 : Constant  Value=Udc*DIODE_D1331SH.Irrm
  D5_4 : Scope
  Data Type Conversion{,1..3,5..6} (6 alike) : DataTypeConversion  OutDataTypeStr=boolean  SaturateOnIntegerOverflow=off  RndMeth=Floor
  Gain42 : Gain  Gain=-1
  Gain43 : Gain  Gain=-1
  Gain46 : Gain
  Gain47 : Gain
  Gain54 : Gain  Gain=0
  Gain55 : Gain
  Gain9 : Gain  Gain=-DIODE_D1331SH.Irrm
  Logical Operator6 : Logic  AllPortsSameDT=off  OutDataTypeStr=boolean
  Logical Operator7 : Logic  AllPortsSameDT=off  OutDataTypeStr=boolean
  Mean{7,69,90,102} (4 alike) : spsMeanLib/Mean  Freq=2000  Vinit=0  Ts=Ts1
  Mean{6,8,68,70,72,91..92,110} (8 alike) : spsMeanLib/Mean  Freq=f  Vinit=0  Ts=Ts1
  Mean71 : spsMeanLib/Mean  Freq=1  Vinit=0  Ts=Ts1
  Mean89 : spsMeanLib/Mean  Freq=f  Vinit=0  Ts=1e-6
  Relational Operator6 : RelationalOperator  Operator=>  OutDataTypeStr=boolean  RndMeth=Simplest  InputSameDT=off
  Relational Operator7 : RelationalOperator  Operator=>  OutDataTypeStr=boolean  RndMeth=Simplest  InputSameDT=off
  Saturation17 : Saturate  UpperLimit=5500  LowerLimit=0
  Saturation19 : Saturate  UpperLimit=5000  LowerLimit=0
  Saturation22 : Saturate  UpperLimit=5500  LowerLimit=0
  Subsystem : Subsystem
  Subsystem1 : Subsystem
  Subsystem2 : Subsystem
  Subsystem29 : Subsystem
  Subsystem3 : Subsystem
  Subsystem34 : Subsystem
  Subsystem4 : Subsystem
  Subsystem5 : Subsystem
  Subsystem53 : Subsystem
  Subsystem6 : Subsystem
  Subsystem8 : Subsystem
  Subsystem9 : Subsystem
  Switch{24..25,33,35..37} (6 alike) : Switch  Criteria=u2 > Threshold  SaturateOnIntegerOverflow=off  InputSameDT=off
  D1_TEMP : Outport
  D1_LOSS_MEAN : Outport  Port=2
  D1_AVG_MEAN : Outport  Port=3
  D1_AVG : Outport  Port=4
  D1_SW_MEAN : Outport  Port=5
  D1_SW : Outport  Port=6
  D2_TEMP : Outport  Port=7
  D2_LOSS_MEAN : Outport  Port=8
  D2_AVG_MEAN : Outport  Port=9
  D2_AVG : Outport  Port=10
  D2_SW_MEAN : Outport  Port=11
  D2_SW : Outport  Port=12
  D5_TEMP : Outport  Port=13
  D5_LOSS_MEAN : Outport  Port=14
  D5_LOSS : Outport  Port=15
  D5_AVG_MEAN : Outport  Port=16
  D5_AVG : Outport  Port=17
  D5_SW_MEAN : Outport  Port=18
  D5_SW : Outport  Port=19
  D7_TEMP : Outport  Port=20
  D7_LOSS_MEAN : Outport  Port=21
  D7_LOSS : Outport  Port=22
  wires:
  Add1/1 -> D2_LOSS_MEAN/1  "D2_LOSS_MEAN"
  Add/1 -> D1_LOSS_MEAN/1  "D1_LOSS_MEAN"
  Add27/1 -> D2_TEMP/1  "D2_TEMP"
  Add4/1 -> D7_TEMP/1  "D7_TEMP"
  U_D7/1 -> Gain9/1
  Mean70/1 -> D5_SW_MEAN/1  "D5_SW_MEAN"
  Subsystem/2(Out2) -> Add41/3
  Saturation17/1 -> Subsystem/1(In1)
  Constant60/1 -> Relational Operator7/2
  Gain47/1 -> Gain43/1
  Data Type Conversion6/1 -> Bitwise Operator18/1
  Constant78/1 -> Relational Operator6/2
  Data Type Conversion5/1 -> Bitwise Operator14/1
  Constant57/1 -> Switch25/1
  Bitwise Operator18/1 -> Logical Operator6/2
  Constant77/1 -> Switch35/3
  Mean89/1 -> Add1/1, D2_AVG_MEAN/1  "D2_AVG_MEAN"
  Subsystem53/1(Out1) -> Add25/2
  Constant52/1 -> Add25/1
  Add43/1 -> D5_TEMP/1  "D5_TEMP"
  Logical Operator6/1 -> Switch33/2
  Constant49/1 -> Switch35/1
  Gain46/1 -> Subsystem29/1(In1)
  Gain42/1 -> Switch24/1, Gain54/1, Relational Operator7/1
  Switch24/1 -> Saturation22/1
  Constant79/1 -> Switch33/3
  Mean92/1 -> Add/1, D1_AVG_MEAN/1  "D1_AVG_MEAN"
  Switch35/1 -> Add41/1
  Switch25/1 -> Add29/1
  Mean6/1 -> D7_LOSS_MEAN/1  "D7_LOSS_MEAN"
  Gain43/1 -> Relational Operator6/1, Gain46/1, Switch33/1
  Add41/1 -> Mean92/1, Subsystem53/1(In1), D1_AVG/1  "D1_AVG"
  Subsystem9/1(Out1) -> Add27/2
  Data Type Conversion2/1 -> Bitwise Operator19/1
  Constant55/1 -> Switch36/3
  Subsystem3/1(Out1) -> Mean7/1
  Subsystem8/2(Out2) -> Add29/3
  Switch37/1 -> Add42/1, Mean71/1
  Constant54/1 -> Switch37/3
  Subsystem5/1(Out1) -> Add43/2
  Subsystem/1(Out1) -> Add41/2
  Gain9/1 -> Add5/1
  Constant58/1 -> Add27/1
  Subsystem4/1(Out1) -> Add42/2
  Mean8/1 -> 34L4520_D1_SW1/1
  Gain54/1 -> Subsystem2/1(In1)
  Mean102/1 -> Subsystem53/2(In2), D1_SW/1, Mean110/1  "D1_SW"
  Subsystem1/1(Out1) -> Add4/2
  Subsystem2/1(Out1) -> Mean90/1
  I_D7/1 -> Subsystem6/1(In1), Subsystem3/1(In1)
  Logical Operator7/1 -> Switch24/2
  Add5/1 -> Subsystem1/1(In1), D7_LOSS/1, Mean6/1  "D7_LOSS"
  Data Type Conversion3/1 -> Bitwise Operator20/2
  Mean7/1 -> Mean8/1, 34L4520_D1_SW1/2
  Relational Operator7/1 -> Logical Operator7/1
  Constant17/1 -> Subsystem1/2(In2)
  Subsystem6/2(Out2) -> Add5/3
  Add25/1 -> D1_TEMP/1  "D1_TEMP"
  Mean69/1 -> Mean70/1, Subsystem5/2(In2), Add28/2, D5_SW/1  "D5_SW"
  Bitwise Operator20/1 -> Switch37/2
  PWM4/1 -> Subsystem34/3(In3)
  Bitwise Operator19/1 -> Switch36/2
  Mean91/1 -> Add1/2, D2_SW_MEAN/1  "D2_SW_MEAN"
  PWM2/1 -> Switch25/2, Data Type Conversion3/1, Data Type Conversion2/1
  Switch33/1 -> Saturation17/1
  Mean110/1 -> Add/2, D1_SW_MEAN/1  "D1_SW_MEAN"
  Mean71/1 -> D5_4/1
  PWM3/1 -> Subsystem2/2(In2), Data Type Conversion5/1, Subsystem29/2(In2), Data Type Conversion6/1, Data Type Conversion1/1
  i/1 -> Gain47/1, Gain55/1, Saturation19/1
  Subsystem8/1(Out1) -> Add29/2
  Data Type Conversion1/1 -> Bitwise Operator19/2
  Constant61/1 -> Switch24/3
  Mean72/1 -> D5_LOSS_MEAN/1  "D5_LOSS_MEAN"
  Mean90/1 -> Mean91/1, Subsystem9/2(In2), D2_SW/1  "D2_SW"
  PWM1/1 -> Switch35/2, Data Type Conversion/1, Subsystem34/2(In2)
  Relational Operator6/1 -> Logical Operator6/1
  Mean68/1 -> D5_AVG_MEAN/1  "D5_AVG_MEAN"
  Saturation19/1 -> Subsystem34/1(In1), Switch36/1
  Switch36/1 -> Subsystem4/1(In1)
  Subsystem4/2(Out2) -> Add42/3
  Gain55/1 -> Gain42/1
  Constant3/1 -> Switch25/3
  Constant9/1 -> Add4/1
  Subsystem34/1(Out1) -> Mean69/1
  Add42/1 -> Mean68/1, Subsystem5/1(In1), Add28/1, D5_AVG/1  "D5_AVG"
  Data Type Conversion/1 -> Bitwise Operator20/1
  Bitwise Operator14/1 -> Logical Operator7/2
  Saturation22/1 -> Subsystem8/1(In1)
  Add29/1 -> Subsystem9/1(In1), D2_AVG/1, Mean89/1  "D2_AVG"
  Constant2/1 -> Switch37/1
  Constant56/1 -> Add43/1
  Subsystem6/1(Out1) -> Add5/2
  Subsystem29/1(Out1) -> Mean102/1
  Add28/1 -> Mean72/1, D5_LOSS/1  "D5_LOSS"

== system igct_diode/IGCT/36L4520/Subsystem ==
  note: T2
  note: T1
  i : Inport
  pwm1 : Inport  Port=2
  pwm2 : Inport  Port=3
  Add26 : Sum
  Add38 : Sum
  Constant1 : Constant  Value=Udc*IGCT_364520_36.Idrm
  Constant50 : Constant  Value=Udc*IGCT_364520_36.Idrm
  Gain50 : Gain
  Gain52 : Gain
  Mean{1,64..65,98} (4 alike) : spsMeanLib/Mean  Freq=f  Vinit=0  Ts=Ts2
  Mean100 : spsMeanLib/Mean  Freq=f  Vinit=0  Ts=Ts1
  Mean{62..63,87,97} (4 alike) : spsMeanLib/Mean  Freq=2000  Vinit=0  Ts=Ts1
  Mean66 : spsMeanLib/Mean  Freq=f  Vinit=0  Ts=Ts1
  Saturation18 : Saturate  UpperLimit=5500  LowerLimit=0
  Saturation23 : Saturate  UpperLimit=5500  LowerLimit=0
  Subsystem1 : Subsystem
  Subsystem2 : Subsystem
  Subsystem31 : Subsystem
  Subsystem56 : Subsystem
  Switch26 : Switch  Criteria=u2 > Threshold  SaturateOnIntegerOverflow=off  InputSameDT=off
  Switch34 : Switch  Criteria=u2 > Threshold  SaturateOnIntegerOverflow=off  InputSameDT=off
  导通损耗 : Subsystem
  导通损耗1 : Subsystem
  T1_TEMP : Outport
  T1_LOSS_MEAN : Outport  Port=2
  T1_LOSS : Outport  Port=3
  T1_AVG_MEAN : Outport  Port=4
  T1_AVG : Outport  Port=5
  T1_SW_MEAN : Outport  Port=6
  T1_SW : Outport  Port=7
  T2_TEMP : Outport  Port=8
  T2_LOSS_MEAN : Outport  Port=9
  T2_LOSS : Outport  Port=10
  T2_AVG_MEAN : Outport  Port=11
  T2_AVG : Outport  Port=12
  T2_SW_MEAN : Outport  Port=13
  T2_SW : Outport  Port=14
  wires:
  Mean87/1 -> Subsystem2/2(SW), Add38/2, T2_SW/1, Mean1/1
  Mean1/1 -> T2_SW_MEAN/1
  Mean66/1 -> T1_LOSS_MEAN/1
  Constant1/1 -> Switch26/3
  Subsystem56/1(PS) -> Mean62/1
  Switch34/1 -> Mean63/1
  Mean63/1 -> Subsystem31/1(AVG), Add26/1, Mean64/1, T1_AVG/1
  Gain52/1 -> Subsystem56/1(I)
  Mean100/1 -> T2_LOSS_MEAN/1
  Add38/1 -> Mean100/1, T2_LOSS/1
  Mean64/1 -> T1_AVG_MEAN/1
  Switch26/1 -> Mean97/1
  Mean98/1 -> T2_AVG_MEAN/1
  Subsystem1/1(PS) -> Mean87/1
  Subsystem2/1(TEMP) -> T2_TEMP/1
  pwm2/1 -> Subsystem1/2(pwm), Switch26/2
  Constant50/1 -> Switch34/3
  Mean97/1 -> Subsystem2/1(AVG), Add38/1, Mean98/1, T2_AVG/1
  Subsystem31/1(TEMP) -> T1_TEMP/1
  Add26/1 -> Mean66/1, T1_LOSS/1
  Mean65/1 -> T1_SW_MEAN/1
  导通损耗1/1(PD) -> Switch26/1
  导通损耗/1(PD) -> Switch34/1
  Mean62/1 -> Subsystem31/2(SW), Add26/2, Mean65/1, T1_SW/1
  pwm1/1 -> Subsystem56/2(pwm), Switch34/2
  Gain50/1 -> Saturation18/1
  Saturation18/1 -> Gain52/1, 导通损耗/1(I)
  i/1 -> Gain50/1, Saturation23/1
  Saturation23/1 -> 导通损耗1/1(I), Subsystem1/1(I)

== system igct_diode/IGCT/36L4521/Subsystem ==
  note: T1
  note: T2
  note: 4522 6KA T2 1.39V 0.39mΩ 3J 21.5J
  note: 4522 6KA T1 1.39V 0.39mΩ 3J 21.5J
  i : Inport
  pwm1 : Inport  Port=2
  pwm2 : Inport  Port=3
  Add26 : Sum
  Add38 : Sum
  Constant1 : Constant  Value=Udc*IGCT_654522_6.Idrm
  Constant50 : Constant  Value=Udc*IGCT_364521_36.Idrm
  Gain50 : Gain
  Gain52 : Gain
  Mean{1,64..65,98} (4 alike) : spsMeanLib/Mean  Freq=f  Vinit=0  Ts=Ts2
  Mean100 : spsMeanLib/Mean  Freq=f  Vinit=0  Ts=Ts1
  Mean{62..63,87,97} (4 alike) : spsMeanLib/Mean  Freq=2000  Vinit=0  Ts=Ts1
  Mean66 : spsMeanLib/Mean  Freq=f  Vinit=0  Ts=Ts1
  Saturation18 : Saturate  UpperLimit=5500  LowerLimit=0
  Saturation23 : Saturate  UpperLimit=5500  LowerLimit=0
  Subsystem1 : Subsystem
  Subsystem2 : Subsystem
  Subsystem31 : Subsystem
  Subsystem56 : Subsystem
  Switch26 : Switch  Criteria=u2 > Threshold  SaturateOnIntegerOverflow=off  InputSameDT=off
  Switch34 : Switch  Criteria=u2 > Threshold  SaturateOnIntegerOverflow=off  InputSameDT=off
  导通损耗 : Subsystem
  导通损耗1 : Subsystem
  T1_TEMP : Outport
  T1_LOSS_MEAN : Outport  Port=2
  T1_LOSS : Outport  Port=3
  T1_AVG_MEAN : Outport  Port=4
  T1_AVG : Outport  Port=5
  T1_SW_MEAN : Outport  Port=6
  T1_SW : Outport  Port=7
  T2_TEMP : Outport  Port=8
  T2_LOSS_MEAN : Outport  Port=9
  T2_LOSS : Outport  Port=10
  T2_AVG_MEAN : Outport  Port=11
  T2_AVG : Outport  Port=12
  T2_SW_MEAN : Outport  Port=13
  T2_SW : Outport  Port=14
  wires:
  Saturation23/1 -> Subsystem1/1(I), 导通损耗1/1(I)
  i/1 -> Saturation23/1, Gain50/1
  Saturation18/1 -> 导通损耗/1(I), Gain52/1
  Gain50/1 -> Saturation18/1
  pwm1/1 -> Switch34/2, Subsystem56/2(pwm)
  Mean62/1 -> T1_SW/1, Mean65/1, Add26/2, Subsystem31/2(SW)
  导通损耗/1(PD) -> Switch34/1
  导通损耗1/1(PD) -> Switch26/1
  Mean65/1 -> T1_SW_MEAN/1
  Add26/1 -> T1_LOSS/1, Mean66/1
  Subsystem31/1(TEMP) -> T1_TEMP/1
  Mean97/1 -> T2_AVG/1, Mean98/1, Subsystem2/1(AVG), Add38/1
  Constant50/1 -> Switch34/3
  pwm2/1 -> Subsystem1/2(pwm), Switch26/2
  Subsystem2/1(TEMP) -> T2_TEMP/1
  Subsystem1/1(PS) -> Mean87/1
  Mean98/1 -> T2_AVG_MEAN/1
  Switch26/1 -> Mean97/1
  Mean64/1 -> T1_AVG_MEAN/1
  Add38/1 -> T2_LOSS/1, Mean100/1
  Mean100/1 -> T2_LOSS_MEAN/1
  Gain52/1 -> Subsystem56/1(I)
  Mean63/1 -> T1_AVG/1, Mean64/1, Add26/1, Subsystem31/1(AVG)
  Switch34/1 -> Mean63/1
  Subsystem56/1(PS) -> Mean62/1
  Constant1/1 -> Switch26/3
  Mean66/1 -> T1_LOSS_MEAN/1
  Mean1/1 -> T2_SW_MEAN/1
  Mean87/1 -> Mean1/1, T2_SW/1, Subsystem2/2(SW), Add38/2

== system igct_diode/IGCT/65L4522/Subsystem ==
  note: T1
  note: T2
  note: 4522 6KA T2 1.39V 0.39mΩ 3J 21.5J
  note: 4522 6KA T1 1.39V 0.39mΩ 3J 21.5J
  i : Inport
  pwm1 : Inport  Port=2
  pwm2 : Inport  Port=3
  Add26 : Sum
  Add38 : Sum
  Constant1 : Constant  Value=Udc*IGCT_654522_6.Idrm
  Constant50 : Constant  Value=Udc*IGCT_654522_6.Idrm
  Gain50 : Gain
  Gain52 : Gain
  Mean{1,64..65,98} (4 alike) : spsMeanLib/Mean  Freq=f  Vinit=0  Ts=Ts2
  Mean100 : spsMeanLib/Mean  Freq=f  Vinit=0  Ts=Ts1
  Mean{62..63,87,97} (4 alike) : spsMeanLib/Mean  Freq=2000  Vinit=0  Ts=Ts1
  Mean66 : spsMeanLib/Mean  Freq=f  Vinit=0  Ts=Ts1
  Saturation18 : Saturate  UpperLimit=5500  LowerLimit=0
  Saturation23 : Saturate  UpperLimit=5500  LowerLimit=0
  Subsystem1 : Subsystem
  Subsystem2 : Subsystem
  Subsystem31 : Subsystem
  Subsystem56 : Subsystem
  Switch26 : Switch  Criteria=u2 > Threshold  SaturateOnIntegerOverflow=off  InputSameDT=off
  Switch34 : Switch  Criteria=u2 > Threshold  SaturateOnIntegerOverflow=off  InputSameDT=off
  导通损耗 : Subsystem
  导通损耗1 : Subsystem
  T1_TEMP : Outport
  T1_LOSS_MEAN : Outport  Port=2
  T1_LOSS : Outport  Port=3
  T1_AVG_MEAN : Outport  Port=4
  T1_AVG : Outport  Port=5
  T1_SW_MEAN : Outport  Port=6
  T1_SW : Outport  Port=7
  T2_TEMP : Outport  Port=8
  T2_LOSS_MEAN : Outport  Port=9
  T2_LOSS : Outport  Port=10
  T2_AVG_MEAN : Outport  Port=11
  T2_AVG : Outport  Port=12
  T2_SW_MEAN : Outport  Port=13
  T2_SW : Outport  Port=14
  wires:
  Saturation23/1 -> Subsystem1/1(I), 导通损耗1/1(I)
  i/1 -> Saturation23/1, Gain50/1
  Saturation18/1 -> 导通损耗/1(I), Gain52/1
  Gain50/1 -> Saturation18/1
  pwm1/1 -> Switch34/2, Subsystem56/2(pwm)
  Mean62/1 -> T1_SW/1, Mean65/1, Add26/2, Subsystem31/2(SW)
  导通损耗/1(PD) -> Switch34/1
  导通损耗1/1(PD) -> Switch26/1
  Mean65/1 -> T1_SW_MEAN/1
  Add26/1 -> T1_LOSS/1, Mean66/1
  Subsystem31/1(TEMP) -> T1_TEMP/1
  Mean97/1 -> T2_AVG/1, Mean98/1, Add38/1, Subsystem2/1(AVG)
  Constant50/1 -> Switch34/3
  pwm2/1 -> Subsystem1/2(pwm), Switch26/2
  Subsystem2/1(TEMP) -> T2_TEMP/1
  Subsystem1/1(PS) -> Mean87/1
  Mean98/1 -> T2_AVG_MEAN/1
  Switch26/1 -> Mean97/1
  Mean64/1 -> T1_AVG_MEAN/1
  Add38/1 -> T2_LOSS/1, Mean100/1
  Mean100/1 -> T2_LOSS_MEAN/1
  Gain52/1 -> Subsystem56/1(I)
  Mean63/1 -> T1_AVG/1, Mean64/1, Add26/1, Subsystem31/1(AVG)
  Switch34/1 -> Mean63/1
  Subsystem56/1(PS) -> Mean62/1
  Constant1/1 -> Switch26/3
  Mean66/1 -> T1_LOSS_MEAN/1
  Mean1/1 -> T2_SW_MEAN/1
  Mean87/1 -> Mean1/1, T2_SW/1, Add38/2, Subsystem2/2(SW)

== system igct_diode/diode_base/base_MAIN/Subsystem ==
  In1 : Inport
  Gain44 : Gain  Gain=b.rF
  Gain45 : Gain  Gain=b.VF0
  Math Function9 : Math  Operator=magnitude^2  SignedPower=on
  Mean79 : spsMeanLib/Mean  Freq=2000  Vinit=0  Ts=Ts1
  RMS9 : spsRMSLib/RMS  TrueRMS=on  Freq=2000  RMSInit=0  Ts=Ts1
  Out1 : Outport
  Out2 : Outport  Port=2
  wires:
  Gain45/1 -> Out2/1
  In1/1 -> RMS9/1, Mean79/1
  Math Function9/1 -> Gain44/1
  Mean79/1 -> Gain45/1
  Gain44/1 -> Out1/1
  RMS9/1 -> Math Function9/1

== system igct_diode/diode_base/base_MAIN/Subsystem1 ==
  note: 散热器热阻：水到壳
  note: 器件手册热阻：壳到结
  note: 接触热阻：散热器到壳
      | 需考虑单面散热还是双面
      | 时间常数估计的？
  In1 : Inport
  In2 : Inport  Port=2
  Add3 : Sum
  Add4 : Sum  Inputs=5
  Add5 : Sum  Inputs=+++
  Constant : Constant  Value=temp_init
  Discrete Filter1 : DiscreteFilter  Numerator=[Ts2/b.Rth_jc1_dou_tau]  Denominator=[1 (Ts2/b.Rth_jc1_dou_tau)-1]  SampleTime=Ts2
  Discrete Filter2 : DiscreteFilter  Numerator=[Ts2/b.Rth_jc2_dou_tau]  Denominator=[1 (Ts2/b.Rth_jc2_dou_tau)-1]  SampleTime=Ts2
  Discrete Filter3 : DiscreteFilter  Numerator=[Ts2/b.Rth_jc3_dou_tau]  Denominator=[1 (Ts2/b.Rth_jc3_dou_tau)-1]  SampleTime=Ts2
  Discrete Filter4 : DiscreteFilter  Numerator=[Ts2/b.Rth_jc4_dou_tau]  Denominator=[1 (Ts2/b.Rth_jc4_dou_tau)-1]  SampleTime=Ts2
  Discrete Filter5 : DiscreteFilter  Numerator=[Ts2/b.Rth_ch_dou_tau]  Denominator=[1 (Ts2/b.Rth_ch_dou_tau)-1]  SampleTime=Ts2
  Discrete Filter9 : DiscreteFilter  Numerator=[Ts2/Rth_h_tau]  Denominator=[1 (Ts2/Rth_h_tau)-1]  SampleTime=Ts2
  Gain1 : Gain  Gain=b.Rth_jc1_dou
  Gain2 : Gain  Gain=b.Rth_jc2_dou
  Gain3 : Gain  Gain=b.Rth_jc3_dou
  Gain4 : Gain  Gain=b.Rth_jc4_dou
  Gain5 : Gain  Gain=b.Rth_ch_dou
  Gain9 : Gain  Gain=Rth_h
  Out1 : Outport  VectorParamsAs1DForOutWhenUnconnected=off
  wires:
  Discrete Filter4/1 -> Add4/5
  Gain4/1 -> Discrete Filter4/1
  In1/1 -> Add3/1
  Gain2/1 -> Discrete Filter2/1
  Discrete Filter2/1 -> Add4/3
  Add4/1 -> Add5/2
  In2/1 -> Add3/2
  Constant/1 -> Add5/3
  Gain1/1 -> Discrete Filter1/1
  Add5/1 -> Out1/1
  Discrete Filter1/1 -> Add4/2
  Gain5/1 -> Discrete Filter5/1
  Discrete Filter5/1 -> Add4/1
  Gain3/1 -> Discrete Filter3/1
  Discrete Filter3/1 -> Add4/4
  Add3/1 -> Gain3/1, Gain5/1, Gain4/1, Gain9/1, Gain1/1, Gain2/1
  Gain9/1 -> Discrete Filter9/1
  Discrete Filter9/1 -> Add5/1

== system igct_diode/diode_base/base_MAIN/Subsystem2 ==
  In1 : Inport
  Gain44 : Gain  Gain=b.rF
  Gain45 : Gain  Gain=b.VF0
  Math Function9 : Math  Operator=magnitude^2  SignedPower=on
  Mean79 : spsMeanLib/Mean  Freq=2000  Vinit=0  Ts=Ts1
  RMS9 : spsRMSLib/RMS  TrueRMS=on  Freq=2000  RMSInit=0  Ts=Ts1
  Out1 : Outport
  Out2 : Outport  Port=2
  wires:
  RMS9/1 -> Math Function9/1
  Gain44/1 -> Out1/1
  Mean79/1 -> Gain45/1
  Math Function9/1 -> Gain44/1
  In1/1 -> Mean79/1, RMS9/1
  Gain45/1 -> Out2/1

== system igct_diode/diode_base/base_MAIN/Subsystem29 ==
  note: 用于判断D1关断时刻，电流为负时，T3开通就意味着D1关断
  In1 : Inport
  In2 : Inport  Port=2
  Abs1 : Abs  SaturateOnIntegerOverflow=off
  Add : Sum
  Constant1 : Constant  Value=0
  Constant2 : Constant  Value=0
  Gain1 : Gain  Gain=Udc/b.Vdc
  Gain2 : Gain  Gain=b.Err/b.IFQ
  Gain3 : Gain  Gain=1/Ts2
  Gain4 : Gain
  Logical Operator2 : Logic  Operator=NOT  AllPortsSameDT=off  OutDataTypeStr=boolean
  Logical Operator3 : Logic  AllPortsSameDT=off  OutDataTypeStr=boolean
  Logical Operator4 : Logic  AllPortsSameDT=off  OutDataTypeStr=boolean
  Logical Operator5 : Logic  Operator=NOT  AllPortsSameDT=off  OutDataTypeStr=boolean
  Pulse Generator : DiscretePulseGenerator  PulseType=Time based  Period=Ts2  PulseWidth=5
  Saturation : Saturate  UpperLimit=5500  LowerLimit=0
  Saturation1 : Saturate  UpperLimit=100  LowerLimit=0
  Switch2 : Switch  Criteria=u2 > Threshold  SaturateOnIntegerOverflow=off  InputSameDT=off
  Switch3 : Switch  Criteria=u2 > Threshold  SaturateOnIntegerOverflow=off  InputSameDT=off
  Switch4 : Switch  Criteria=u2 > Threshold  SaturateOnIntegerOverflow=off  InputSameDT=off
  Unit Delay{,1..3} (4 alike) : UnitDelay  SampleTime=Ts1  HasFrameUpgradeWarning=on
  Out1 : Outport  VectorParamsAs1DForOutWhenUnconnected=off
  wires:
  Gain2/1 -> Saturation1/1
  Saturation/1 -> Gain2/1
  Saturation1/1 -> Switch2/1
  Gain4/1 -> Saturation/1
  Unit Delay/1 -> Logical Operator2/1
  Add/1 -> Unit Delay1/1
  In1/1 -> Gain4/1
  Gain3/1 -> Out1/1
  Unit Delay1/1 -> Switch4/1, Switch3/3
  Logical Operator4/1 -> Switch3/2, Switch4/2
  Logical Operator5/1 -> Logical Operator4/2
  Unit Delay3/1 -> Logical Operator5/1
  Unit Delay2/1 -> Switch4/3
  Switch4/1 -> Gain3/1, Unit Delay2/1
  Pulse Generator/1 -> Logical Operator4/1, Unit Delay3/1
  Constant1/1 -> Switch3/1
  Switch3/1 -> Add/2
  Constant2/1 -> Switch2/3
  Logical Operator3/1 -> Switch2/2
  Logical Operator2/1 -> Logical Operator3/2
  In2/1 -> Unit Delay/1, Logical Operator3/1
  Gain1/1 -> Abs1/1
  Switch2/1 -> Gain1/1
  Abs1/1 -> Add/1

== system igct_diode/diode_base/base_MAIN/Subsystem3 ==
  In1 : Inport
  Abs1 : Abs  SaturateOnIntegerOverflow=off
  Add : Sum
  Add1 : Sum
  Constant : Constant
  Constant1 : Constant  Value=0
  Constant2 : Constant  Value=0
  Data Type Conversion : DataTypeConversion  OutDataTypeStr=boolean  SaturateOnIntegerOverflow=off  RndMeth=Floor
  Data Type Conversion1 : DataTypeConversion  SaturateOnIntegerOverflow=off  RndMeth=Floor
  Gain : Gain  Gain=-1
  Gain2 : Gain  Gain=Udc/b.Vdc
  Gain3 : Gain  Gain=1/Ts2
  Gain6 : Gain
  Gain8 : Gain  Gain=b.Err/b.IFQ
  Logical Operator2 : Logic  Operator=NOT  AllPortsSameDT=off  OutDataTypeStr=boolean
  Logical Operator4 : Logic  AllPortsSameDT=off  OutDataTypeStr=boolean
  Logical Operator5 : Logic  Operator=NOT  AllPortsSameDT=off  OutDataTypeStr=boolean
  Pulse Generator : DiscretePulseGenerator  PulseType=Time based  Period=Ts2  PulseWidth=5
  Saturation2 : Saturate  UpperLimit=5500  LowerLimit=0
  Saturation3 : Saturate  UpperLimit=100  LowerLimit=0
  Scope1 : Scope  NumInputPorts=3
  Scope7 : Scope  NumInputPorts=2
  Switch2 : Switch  Criteria=u2 > Threshold  Threshold=-1  SaturateOnIntegerOverflow=off  InputSameDT=off
  Switch3 : Switch  Criteria=u2 > Threshold  SaturateOnIntegerOverflow=off  InputSameDT=off
  Switch4 : Switch  Criteria=u2 > Threshold  SaturateOnIntegerOverflow=off  InputSameDT=off
  Terminator : Terminator
  Unit Delay{,1..3} (4 alike) : UnitDelay  SampleTime=1e-6  HasFrameUpgradeWarning=on
  Out1 : Outport  VectorParamsAs1DForOutWhenUnconnected=off
  wires:
  Saturation3/1 -> Terminator/1
  Gain8/1 -> Saturation3/1
  Saturation2/1 -> Gain8/1
  Gain6/1 -> Saturation2/1
  Constant/1 -> Switch2/1
  Data Type Conversion1/1 -> Gain/1
  Gain/1 -> Switch2/2
  Add1/1 -> Data Type Conversion1/1
  Data Type Conversion/1 -> Unit Delay/1, Add1/1
  Logical Operator2/1 -> Add1/2
  Unit Delay/1 -> Logical Operator2/1
  Abs1/1 -> Add/1
  Switch2/1 -> Gain2/1
  Gain2/1 -> Abs1/1, Scope1/1
  In1/1 -> Gain6/1, Data Type Conversion/1
  Constant2/1 -> Switch2/3
  Switch3/1 -> Add/2
  Constant1/1 -> Switch3/1
  Pulse Generator/1 -> Unit Delay3/1, Logical Operator4/1
  Switch4/1 -> Scope7/2, Unit Delay2/1, Gain3/1
  Unit Delay2/1 -> Switch4/3
  Unit Delay3/1 -> Logical Operator5/1
  Logical Operator5/1 -> Logical Operator4/2
  Logical Operator4/1 -> Scope1/3, Switch4/2, Switch3/2
  Unit Delay1/1 -> Scope7/1, Switch3/3, Switch4/1
  Gain3/1 -> Out1/1
  Add/1 -> Scope1/2, Unit Delay1/1

== system igct_diode/diode_base/base_MAIN/Subsystem34 ==
  In1 : Inport
  In2 : Inport  Port=2
  In3 : Inport  Port=3
  Abs1 : Abs  SaturateOnIntegerOverflow=off
  Add : Sum
  Constant1 : Constant  Value=0
  Constant2 : Constant  Value=0
  Gain2 : Gain  Gain=Udc/b.Vdc
  Gain3 : Gain  Gain=1/Ts2
  Gain4 : Gain
  Gain8 : Gain  Gain=b.Err/b.IFQ
  Logical Operator1 : Logic  Operator=NOT  AllPortsSameDT=off  OutDataTypeStr=boolean
  Logical Operator11 : Logic  Operator=OR  AllPortsSameDT=off  OutDataTypeStr=boolean
  Logical Operator2 : Logic  Operator=NOT  AllPortsSameDT=off  OutDataTypeStr=boolean
  Logical Operator3 : Logic  AllPortsSameDT=off  OutDataTypeStr=boolean
  Logical Operator4 : Logic  AllPortsSameDT=off  OutDataTypeStr=boolean
  Logical Operator5 : Logic  Operator=NOT  AllPortsSameDT=off  OutDataTypeStr=boolean
  Logical Operator6 : Logic  AllPortsSameDT=off  OutDataTypeStr=boolean
  Pulse Generator : DiscretePulseGenerator  PulseType=Time based  Period=Ts2  PulseWidth=5
  Saturation : Saturate  UpperLimit=5500  LowerLimit=0
  Saturation1 : Saturate  UpperLimit=100  LowerLimit=0
  Scope1 : Scope  NumInputPorts=3
  Scope7 : Scope  NumInputPorts=2
  Switch2 : Switch  Criteria=u2 > Threshold  SaturateOnIntegerOverflow=off  InputSameDT=off
  Switch3 : Switch  Criteria=u2 > Threshold  SaturateOnIntegerOverflow=off  InputSameDT=off
  Switch4 : Switch  Criteria=u2 > Threshold  SaturateOnIntegerOverflow=off  InputSameDT=off
  Unit Delay{,1..4} (5 alike) : UnitDelay  SampleTime=1e-6  HasFrameUpgradeWarning=on
  Out1 : Outport  VectorParamsAs1DForOutWhenUnconnected=off
  wires:
  Gain8/1 -> Saturation1/1
  Saturation/1 -> Gain8/1
  Logical Operator3/1 -> Logical Operator11/1
  Logical Operator11/1 -> Switch2/2
  Logical Operator1/1 -> Logical Operator6/2
  Logical Operator6/1 -> Logical Operator11/2
  Unit Delay4/1 -> Logical Operator1/1
  In3/1 -> Logical Operator6/1, Unit Delay4/1
  Saturation1/1 -> Switch2/1
  Gain4/1 -> Saturation/1
  Unit Delay/1 -> Logical Operator2/1
  Add/1 -> Unit Delay1/1, Scope1/2
  In1/1 -> Gain4/1
  Gain3/1 -> Out1/1
  Unit Delay1/1 -> Switch3/3, Switch4/1, Scope7/1
  Logical Operator4/1 -> Scope1/3, Switch3/2, Switch4/2
  Logical Operator5/1 -> Logical Operator4/2
  Unit Delay3/1 -> Logical Operator5/1
  Unit Delay2/1 -> Switch4/3
  Switch4/1 -> Unit Delay2/1, Gain3/1, Scope7/2
  Pulse Generator/1 -> Logical Operator4/1, Unit Delay3/1
  Constant1/1 -> Switch3/1
  Switch3/1 -> Add/2
  Constant2/1 -> Switch2/3
  Logical Operator2/1 -> Logical Operator3/2
  In2/1 -> Unit Delay/1, Logical Operator3/1
  Gain2/1 -> Scope1/1, Abs1/1
  Switch2/1 -> Gain2/1
  Abs1/1 -> Add/1

== system igct_diode/diode_base/base_MAIN/Subsystem4 ==
  In1 : Inport
  Gain44 : Gain  Gain=b.rF
  Gain45 : Gain  Gain=b.VF0
  Math Function9 : Math  Operator=magnitude^2  SignedPower=on
  Mean79 : spsMeanLib/Mean  Freq=2000  Vinit=0  Ts=Ts1
  RMS9 : spsRMSLib/RMS  TrueRMS=on  Freq=2000  RMSInit=0  Ts=Ts1
  Out1 : Outport
  Out2 : Outport  Port=2
  wires:
  RMS9/1 -> Math Function9/1
  Gain44/1 -> Out1/1
  Mean79/1 -> Gain45/1
  Math Function9/1 -> Gain44/1
  In1/1 -> Mean79/1, RMS9/1
  Gain45/1 -> Out2/1

== system igct_diode/diode_base/base_MAIN/Subsystem5 ==
  note: 用于判断D1关断时刻，电流为负时，T3开通就意味着D1关断
  In1 : Inport
  In2 : Inport  Port=2
  Abs1 : Abs  SaturateOnIntegerOverflow=off
  Add : Sum
  Constant1 : Constant  Value=0
  Constant2 : Constant  Value=0
  Gain1 : Gain  Gain=Udc/b.Vdc
  Gain2 : Gain  Gain=b.Err/b.IFQ
  Gain3 : Gain  Gain=1/Ts2
  Gain4 : Gain
  Logical Operator2 : Logic  Operator=NOT  AllPortsSameDT=off  OutDataTypeStr=boolean
  Logical Operator3 : Logic  AllPortsSameDT=off  OutDataTypeStr=boolean
  Logical Operator4 : Logic  AllPortsSameDT=off  OutDataTypeStr=boolean
  Logical Operator5 : Logic  Operator=NOT  AllPortsSameDT=off  OutDataTypeStr=boolean
  Pulse Generator : DiscretePulseGenerator  PulseType=Time based  Period=Ts2  PulseWidth=5
  Saturation : Saturate  UpperLimit=5500  LowerLimit=0
  Saturation1 : Saturate  UpperLimit=100  LowerLimit=0
  Switch2 : Switch  Criteria=u2 > Threshold  SaturateOnIntegerOverflow=off  InputSameDT=off
  Switch3 : Switch  Criteria=u2 > Threshold  SaturateOnIntegerOverflow=off  InputSameDT=off
  Switch4 : Switch  Criteria=u2 > Threshold  SaturateOnIntegerOverflow=off  InputSameDT=off
  Unit Delay{,1..3} (4 alike) : UnitDelay  SampleTime=Ts1  HasFrameUpgradeWarning=on
  Out1 : Outport  VectorParamsAs1DForOutWhenUnconnected=off
  wires:
  Abs1/1 -> Add/1
  Switch2/1 -> Gain1/1
  Gain1/1 -> Abs1/1
  In2/1 -> Logical Operator3/1, Unit Delay/1
  Logical Operator2/1 -> Logical Operator3/2
  Logical Operator3/1 -> Switch2/2
  Constant2/1 -> Switch2/3
  Switch3/1 -> Add/2
  Constant1/1 -> Switch3/1
  Pulse Generator/1 -> Unit Delay3/1, Logical Operator4/1
  Switch4/1 -> Unit Delay2/1, Gain3/1
  Unit Delay2/1 -> Switch4/3
  Unit Delay3/1 -> Logical Operator5/1
  Logical Operator5/1 -> Logical Operator4/2
  Logical Operator4/1 -> Switch4/2, Switch3/2
  Unit Delay1/1 -> Switch3/3, Switch4/1
  Gain3/1 -> Out1/1
  In1/1 -> Gain4/1
  Add/1 -> Unit Delay1/1
  Unit Delay/1 -> Logical Operator2/1
  Gain4/1 -> Saturation/1
  Saturation1/1 -> Switch2/1
  Saturation/1 -> Gain2/1
  Gain2/1 -> Saturation1/1
